simulink model "ReadyModels"  (R2025b)
settings: Solver=VariableStepAuto  StartTime=0.0  StopTime=10  RelTol=1e-3
model workspace (MAT data in the model file):
  Kt = 0.04
undefined symbols (not defined in the file): Ion, Lithium
libraries: spsDiodeLib x4, spsVoltageMeasurementLib x4, spsCurrentMeasurementLib x3, spsSeriesRLCBranchLib x3, spsBatteryLib x1, spsBoostConverterLib x1, spsDCMachineLib x1, spsGroundLib x1, sps_lib x1
settings Model: Creator=khalid  LastModifiedBy=khalidwaleed

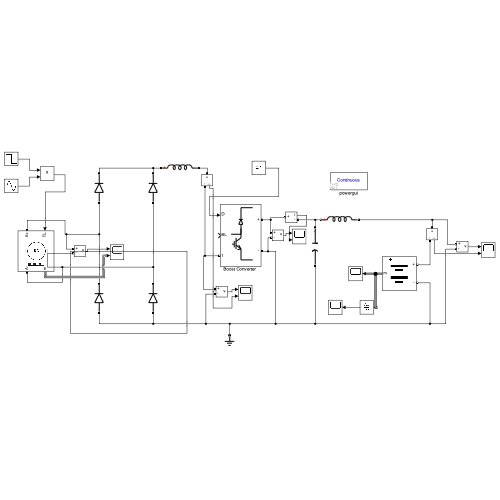
[thumbnail: Simulink's stored preview of the top-level diagram]
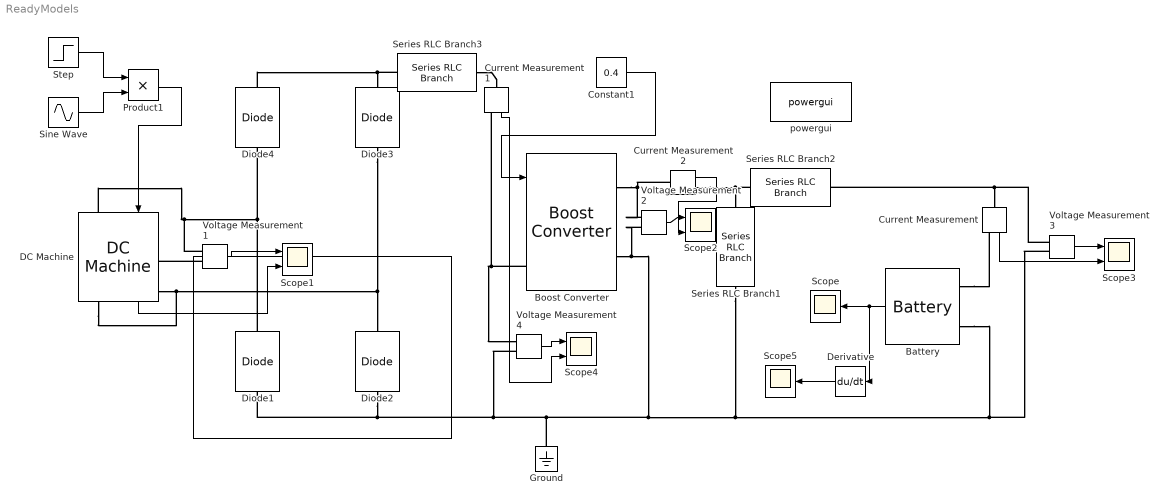
== system ReadyModels ==
  Battery : spsBatteryLib/Battery  BatType=Lithium-Ion  NomV=7.2  NomQ=5.4  SOC=0  Batt_Tr=30  PresetModel=on  MaxQ=5.4  MinV=5.4  FullV=8.3807  Dis_rate=2.3478  R=0.013333  Normal_OP=4.8835  expZone="[7.7788      0.2653]"
  "Boost Converter " : spsBoostConverterLib/Boost Converter  ModelType=Average model (D-controlled)  Ron=1e-3  Rs=1e6  Cs=inf  Vforward=[0,0]  Ron_Diode=1e-3  Rs_Diode=1e6  Cs_Diode=inf  Vf_Diode=1e-3  Rs_CurrentSource=inf  Ron_ACsource=1e-3
      settings: LibrarySourceBlock=sps_lib/Power Electronics/Boost Converter
  Constant1 : Constant  Value=0.4
  Current Measurement : spsCurrentMeasurementLib/Current Measurement  PhasorSimulation=off  OutputType=Complex  PSBequivalent=0
  Current Measurement1 : spsCurrentMeasurementLib/Current Measurement  PhasorSimulation=off  OutputType=Complex  PSBequivalent=0
  Current Measurement2 : spsCurrentMeasurementLib/Current Measurement  PhasorSimulation=off  OutputType=Complex  PSBequivalent=0
  DC Machine : spsDCMachineLib/DC Machine  PresetModel=No  MechanicalLoad=Torque TL  FieldType=Permanent magnet  ShowDetailedParameters=on  MeasurementBus=on  RLa="[ 1  0.5]"  RLf="[ 240  120]"  Laf=1.8  MachineConstant=Back-emf constant (V/rpm)  Ke=0.1  Kt=1.8  J=0.01  Bm=0.1  Tf=0  w0=0  Ifinit=1  TsPowergui=0  TsBlock=-1
  Derivative : Derivative
  Diode{1..4} (4 alike) : spsDiodeLib/Diode  Ron=0.001  Lon=0  Vf=0.8  IC=0  UseSnubber=0  Rs=0  Cs=0  Measurements=off
  Ground : spsGroundLib/Ground  LConnTagsString=a
  Product1 : Product
  Scope : Scope
      settings: ActiveDisplayYMinimum=3.2787807508978233  ActiveDisplayYMaximum=3.37269021788256  DataLoggingVariableName=ScopeData4
  Scope{1..4} (4 alike) : Scope  NumInputPorts=2
      Scope1 settings: ActiveDisplayYMinimum=-19.598171910042659  ActiveDisplayYMaximum=22.100887689014026
      Scope2 settings: ActiveDisplayYMinimum=-0.82083849483325066  ActiveDisplayYMaximum=7.3875464534978788  DataLoggingVariableName=ScopeData2
      Scope3 settings: ActiveDisplayYMinimum=-0.89465290097761119  ActiveDisplayYMaximum=6.0509199216083944
      Scope4 settings: ActiveDisplayYMinimum=-1.1159152762524198  ActiveDisplayYMaximum=10.043237486271451  DataLoggingVariableName=ScopeData3
  Scope5 : Scope
      settings: ActiveDisplayYMinimum=-159.336  ActiveDisplayYMaximum=78.264  DataLoggingVariableName=ScopeData5
  Series RLC Branch1 : spsSeriesRLCBranchLib/Series RLC Branch  LConnTagsString=__new0  RConnTagsString=__new0  BranchType=C  Resistance=1  Inductance=1e-3  SetiL0=off  InitialCurrent=0  Capacitance=1e-3  Setx0=off  InitialVoltage=0  Measurements=None
  Series RLC Branch2 : spsSeriesRLCBranchLib/Series RLC Branch  LConnTagsString=__new0  RConnTagsString=__new0  BranchType=L  Resistance=1  Inductance=1e-3  SetiL0=off  InitialCurrent=0  Capacitance=1e-6  Setx0=off  InitialVoltage=0  Measurements=None
  Series RLC Branch3 : spsSeriesRLCBranchLib/Series RLC Branch  LConnTagsString=__new0  RConnTagsString=__new0  BranchType=L  Resistance=1  Inductance=25e-3  SetiL0=off  InitialCurrent=0  Capacitance=1e-6  Setx0=off  InitialVoltage=0  Measurements=None
  Sine Wave : Sin  Amplitude=10  Frequency=4/(2*pi)  SampleTime=0
  Step : Step  Time=4  Before=1  After=0  SampleTime=0
  Voltage Measurement{1..4} (4 alike) : spsVoltageMeasurementLib/Voltage Measurement  PhasorSimulation=off  OutputType=Complex  PSBequivalent=0
  powergui : sps_lib/powergui  Priority=1  SimulationMode=Continuous  SampleTime=50e-6  frequency=60  Iterations=50  frequencyindice=0  Pbase=100e6  ErrMax=1e-4  UnitsV=kV  UnitsW=MW  buscounter=0  FunctionMessages=off  echomessages=off  EnableUseOfTLC=off  CurrentSourceSwitches=off  DisableSnubberDevices=off  DisableRonSwitches=off  DisableVfSwitches=off  DisplayEquations=off  AutomaticDiscreteSolvers=off  SolverType=Tustin/Backward Euler (TBE)  Interpol=off  ExternalGateDelay=off  methode=off  Ts=100  x0status=blocks  SPID=on  SwTol=0  HookPort=off  NonlinearTolerance=1e-4  nMaxIteration=100  ContinueOnMaxIteration=off  RestoreLinks=warning  ResistiveCurrentMeasurement=off  Frange=[0:2:500]  Ylog=off  Xlog=on  ShowGrid=off  save=off  variable=ZData  structure=0  ZoomFFT=off  StartTime=0.0  cycles=1  DisplayStyle=1  fundamental=60  FreqAxis=off  MaxFrequency=1000  frequencyindicesteady=1  RmsSteady=1  display=off
  wires:
  Product1/1 -> DC Machine/1
  Constant1/1 -> "Boost Converter "/1
  Voltage Measurement1/1 -> Scope1/1
  Voltage Measurement2/1 -> Scope2/1
  DC Machine/1 -> Scope1/2
  Voltage Measurement3/1 -> Scope3/1
  Current Measurement/1 -> Scope3/2
  Voltage Measurement4/1 -> Scope4/1
  Current Measurement1/1 -> Scope4/2
  Current Measurement2/1 -> Scope2/2
  Battery/1 -> Derivative/1, Scope/1
  Step/1 -> Product1/1
  Sine Wave/1 -> Product1/2
  Derivative/1 -> Scope5/1
  connections:
  Diode1/RConn1 -- Voltage Measurement1/LConn1 -- DC Machine/LConn1 -- Diode4/LConn1
  Diode3/LConn1 -- Voltage Measurement1/LConn2 -- DC Machine/RConn1 -- Diode2/RConn1
  Diode4/RConn1 -- Series RLC Branch3/LConn1 -- Diode3/RConn1
  Diode2/LConn1 -- Battery/LConn2 -- Voltage Measurement3/LConn2 -- Series RLC Branch1/RConn1 -- "Boost Converter "/RConn2 -- Voltage Measurement2/LConn2 -- Ground/LConn1 -- Voltage Measurement4/LConn2 -- Diode1/LConn1
  Series RLC Branch2/LConn1 -- Series RLC Branch1/LConn1 -- Current Measurement2/RConn1
  Battery/LConn1 -- Current Measurement/RConn1
  Voltage Measurement3/LConn1 -- Series RLC Branch2/RConn1 -- Current Measurement/LConn1
  Current Measurement1/RConn1 -- "Boost Converter "/LConn1 -- Voltage Measurement4/LConn1
  Voltage Measurement2/LConn1 -- "Boost Converter "/RConn1 -- Current Measurement2/LConn1
  Series RLC Branch3/RConn1 -- Current Measurement1/LConn1
